simulink model "hoop_ident"  (R2016b)
settings: Solver=FixedStepAuto  StartTime=0.0  StopTime=15  FixedStep=1/50  RelTol=1e-3
PreLoadFcn:
  | Ts = 1e-3
undefined symbols (not defined in the file or in its folder): prms
libraries: raspi_library x2, simulink x1
PreSaveFcn:
  | set_param(gcs, 'location', [15 50 815 560])
settings Model: SimulationMode=external  Creator=The MathWorks Inc.  LastModifiedBy=marti
settings SolverCC: PositivePriorityOrder=on
settings DataIOCC: LimitDataPoints=on  SaveFormat=Array
settings OptimizationCC: BlockReduction=off  BooleanDataType=off  DefaultUnderspecifiedDataType=single  LifeSpan=inf  MaxStackSize=64
settings DebuggingCC: SaveWithParameterizedLinksMsg=none  UnderspecifiedInitializationDetection=Classic  MergeDetectMultiDrivingBlocksExec=none  SignalResolutionControl=TryResolveAllWithWarning  ParameterTunabilityLossMsg=error  SFUnexpectedBacktrackingDiag=warning  SFNoUnconditionalDefaultTransitionDiag=warning  SFExecutionAtInitializationDiag=none
settings HardwareCC: ProdBitPerPointer=32  ProdBitPerSizeT=32  ProdBitPerPtrDiffT=32  ProdLargestAtomicInteger=Long  ProdLargestAtomicFloat=Double  ProdWordSize=32  ProdHWDeviceType=ARM Compatible->ARM Cortex
settings ModelReferenceCC: PropagateSignalLabelsOutOfModel=off
settings RTWCC: SystemTargetFile=ert.tlc  HardwareBoard=Raspberry Pi  TLCOptions=-aInlineSetEventsForThisBaseRateFcn=TLC_FALSE -aSuppressMultiTaskScheduler=TLC_FALSE -aRateBasedStepFcn=0  TemplateMakefile=ert_default_tmf  Description=Embedded Coder  GenerateReport=on  RTWVerbose=off  Toolchain=GNU GCC Raspberry Pi  BuildConfiguration=Specify  IncludeHyperlinkInReport=on  GenerateTraceInfo=on  GenerateTraceReport=on  GenerateTraceReportSl=on  GenerateTraceReportSf=on  GenerateTraceReportEml=on
settings CodeAppCC: ForceParamTrailComments=on  IgnoreCustomStorageClasses=off  OperatorAnnotations=on  SimulinkDataObjDesc=on  SFDataObjDesc=on  MATLABFcnDesc=on  MangleLength=10  InsertBlockDesc=on  MATLABSourceComments=on
settings ERTTargetCC: SupportVariableSizeSignals=on
settings ConfigComp: CovMetricSettings=dw  CovHtmlReporting=on  CovSaveCumulativeToWorkspaceVar=on  CovSaveSingleToWorkspaceVar=on  CovExternalEMLEnable=off  CovSFcnEnable=off

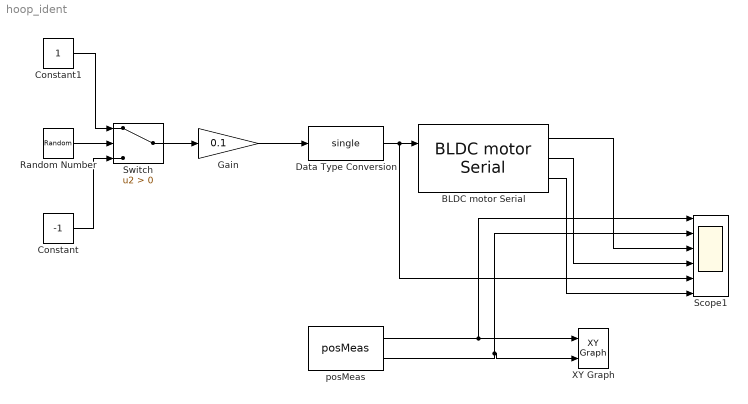
== system hoop_ident ==
  BLDC motor Serial : raspi_library/BLDC motor Serial  sampleTime=prms.Ts
  Constant : Constant  Value=-1
  Constant1 : Constant
  Data Type Conversion : DataTypeConversion  OutDataTypeStr=single
  Gain : Gain  Gain=0.1
  Random Number : RandomNumber  SampleTime=prms.Ts
  Scope1 : Scope  NumInputPorts=6
  Switch : Switch  Criteria=u2 > Threshold
  XY Graph : simulink/Sinks/XY Graph  xmin=0  xmax=480  ymin=0  ymax=480  st=-1
  posMeas : raspi_library/posMeas  sampleTime=1/50
  wires:
  posMeas/2 -> Scope1/2, XY Graph/2
  posMeas/1 -> Scope1/1, XY Graph/1
  Gain/1 -> Data Type Conversion/1
  Data Type Conversion/1 -> Scope1/5, BLDC motor Serial/1
  Switch/1 -> Gain/1
  Random Number/1 -> Switch/2
  Constant/1 -> Switch/3
  Constant1/1 -> Switch/1
  BLDC motor Serial/1 -> Scope1/3
  BLDC motor Serial/2 -> Scope1/4
  BLDC motor Serial/3 -> Scope1/6
